simulink model "ECM_Cell"  (R2025a)
settings: Solver=FixedStepDiscrete  StartTime=0.0  StopTime=1*dt  FixedStep=dt  RelTol=1e-3
values from neighbouring files (symbols this model uses):
  a1_tbl = [ ... (first row only)    [parameters.m]
  a2_tbl = [ ... (first row only)    [parameters.m]
  C1_tbl = [ ... (first row only)    [parameters.m]
  c1_tbl = [ ... (first row only)    [parameters.m]
  C2_tbl = [ ... (first row only)    [parameters.m]
  c2_tbl = [ ... (first row only)    [parameters.m]
  I = 2    [parameters.m]
  I_bp = [1, 2, 3, 4, 5, 6, 7, 8, 9, 10, 11, 12, 13, 14, 15, 16]    [parameters.m]
  R0_tbl = [ ... (first row only)    [parameters.m]
  R1_tbl = [ ... (first row only)    [parameters.m]
  R2_tbl = [ ... (first row only)    [parameters.m]
  SOC_bp = [0, 10, 20, 30, 40, 50, 60, 70, 80, 90, 100]    [parameters.m]
  SOC_init = 80    [parameters.m]
undefined symbols (not defined in the file or in its folder): DiscIntNeverNeededParam
settings Model: Creator=ludvig  LastModifiedBy=ludvig

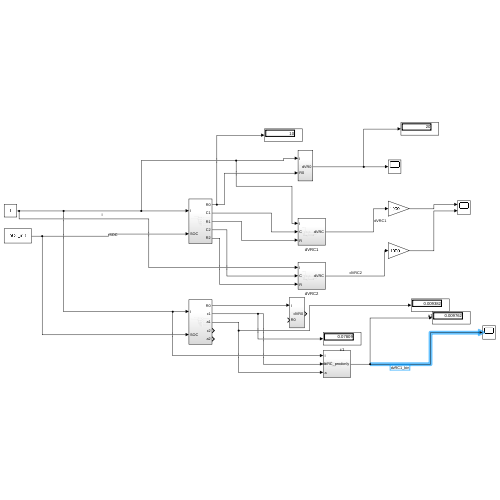
[thumbnail: Simulink's stored preview of the top-level diagram]
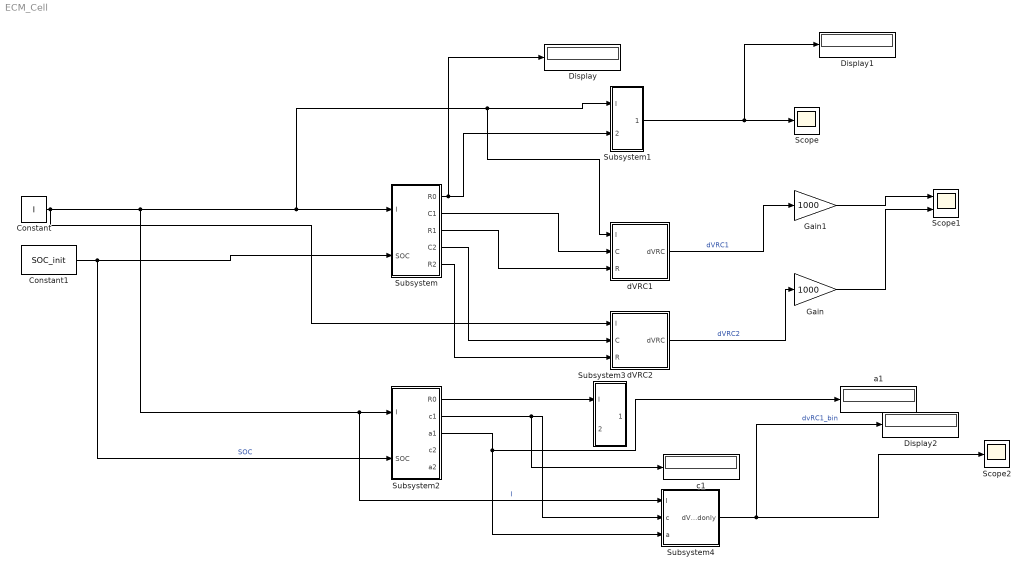
== system ECM_Cell ==
  Constant : Constant  Value=I
  Constant1 : Constant  Value=SOC_init
  Display : Display
  Display1 : Display
  Display2 : Display
  Gain : Gain  Gain=1000
  Gain1 : Gain  Gain=1000
  Scope : Scope
      settings: ActiveDisplayYMinimum=10  ActiveDisplayYMaximum=30
  Scope1 : Scope  NumInputPorts=2
      settings: ActiveDisplayYMinimum=7.0775458763666457  ActiveDisplayYMaximum=30.641709754209629
  Scope2 : Scope
      settings: ActiveDisplayYMinimum=-0.0012202262878417967  ActiveDisplayYMaximum=0.010982036590576172  DataLoggingVariableName=ScopeData2
  Subsystem : Subsystem
  Subsystem1 : Subsystem
  Subsystem2 : Subsystem
  Subsystem3 : Subsystem
  Subsystem4 : Subsystem
  a1 : Display
  c1 : Display
  dVRC1 : Subsystem
  dVRC2 : Subsystem
  wires:
  Constant/1 -> dVRC2/1(I), Subsystem4/1(I), Subsystem2/1(I), dVRC1/1(I), Subsystem1/1(I), Subsystem/1(I)  "I"
  Constant1/1 -> Subsystem2/2(SOC), Subsystem/2(SOC)  "SOC"
  Subsystem/1(R0) -> Display/1, Subsystem1/2(R0)
  Subsystem1/1(dVR0) -> Display1/1, Scope/1
  Subsystem/2(C1) -> dVRC1/2(C)
  Subsystem/3(R1) -> dVRC1/3(R)
  dVRC1/1(dVRC) -> Gain1/1  "dVRC1"
  Subsystem/4(C2) -> dVRC2/2(C)
  Subsystem/5(R2) -> dVRC2/3(R)
  dVRC2/1(dVRC) -> Gain/1  "dVRC2"
  Gain/1 -> Scope1/2
  Gain1/1 -> Scope1/1
  Subsystem2/1(R0) -> Subsystem3/1(I)
  Subsystem2/2(c1) -> c1/1, Subsystem4/2(c)
  Subsystem2/3(a1) -> a1/1, Subsystem4/3(a)
  Subsystem4/1(dVRC_prodonly) -> Display2/1, Scope2/1  "dvRC1_bin"

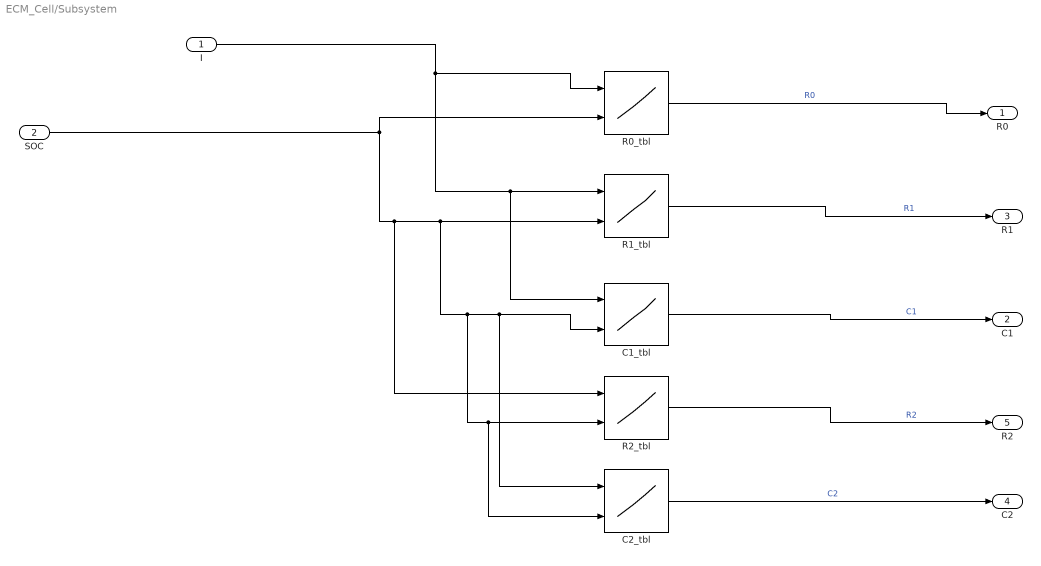
== system ECM_Cell/Subsystem ==
  I : Inport
  SOC : Inport  Port=2
  C1_tbl : Lookup_n-D  BreakpointsForDimension1=I_bp  BreakpointsForDimension2=SOC_bp  Table=C1_tbl  InternalRulePriority=Speed  RndMeth=Simplest
      settings: InputPortMap=u0,u1
  C2_tbl : Lookup_n-D  BreakpointsForDimension1=I_bp  BreakpointsForDimension2=SOC_bp  Table=C2_tbl  InternalRulePriority=Speed  RndMeth=Simplest
      settings: InputPortMap=u0,u1
  R0_tbl : Lookup_n-D  BreakpointsForDimension1=I_bp  BreakpointsForDimension2=SOC_bp  Table=R0_tbl  InternalRulePriority=Speed  RndMeth=Simplest
      settings: InputPortMap=u0,u1
  R1_tbl : Lookup_n-D  BreakpointsForDimension1=I_bp  BreakpointsForDimension2=SOC_bp  Table=R1_tbl  InternalRulePriority=Speed  RndMeth=Simplest
      settings: InputPortMap=u0,u1
  R2_tbl : Lookup_n-D  BreakpointsForDimension1=I_bp  BreakpointsForDimension2=SOC_bp  Table=R2_tbl  InternalRulePriority=Speed  RndMeth=Simplest
      settings: InputPortMap=u0,u1
  R0 : Outport
  C1 : Outport  Port=2
  R1 : Outport  Port=3
  C2 : Outport  Port=4
  R2 : Outport  Port=5
  wires:
  I/1 -> C1_tbl/1, R1_tbl/1, R0_tbl/1
  SOC/1 -> R2_tbl/1, C2_tbl/2, R2_tbl/2, C2_tbl/1, C1_tbl/2, R1_tbl/2, R0_tbl/2
  C1_tbl/1 -> C1/1  "C1"
  C2_tbl/1 -> C2/1  "C2"
  R0_tbl/1 -> R0/1  "R0"
  R2_tbl/1 -> R2/1  "R2"
  R1_tbl/1 -> R1/1  "R1"

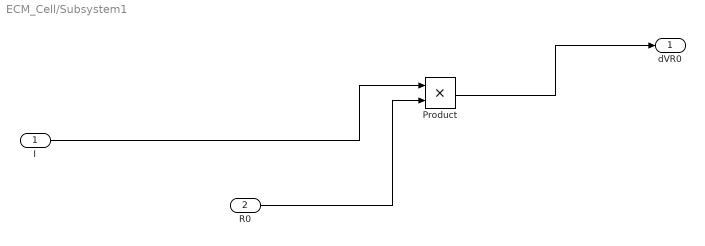
== system ECM_Cell/Subsystem1 ==
  I : Inport
  R0 : Inport  Port=2
  Product : Product
  dVR0 : Outport
  wires:
  Product/1 -> dVR0/1
  I/1 -> Product/1
  R0/1 -> Product/2

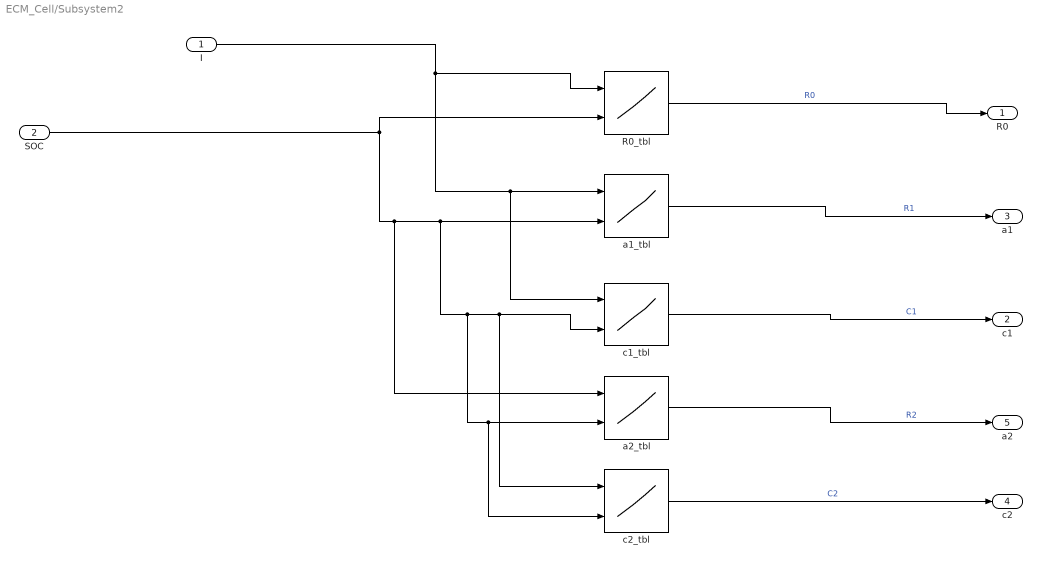
== system ECM_Cell/Subsystem2 ==
  I : Inport
  SOC : Inport  Port=2
  R0_tbl : Lookup_n-D  BreakpointsForDimension1=I_bp  BreakpointsForDimension2=SOC_bp  Table=R0_tbl  InternalRulePriority=Speed  RndMeth=Simplest
      settings: InputPortMap=u0,u1
  a1_tbl : Lookup_n-D  BreakpointsForDimension1=I_bp  BreakpointsForDimension2=SOC_bp  Table=a1_tbl  InternalRulePriority=Speed  RndMeth=Simplest
      settings: InputPortMap=u0,u1
  a2_tbl : Lookup_n-D  BreakpointsForDimension1=I_bp  BreakpointsForDimension2=SOC_bp  Table=a2_tbl  InternalRulePriority=Speed  RndMeth=Simplest
      settings: InputPortMap=u0,u1
  c1_tbl : Lookup_n-D  BreakpointsForDimension1=I_bp  BreakpointsForDimension2=SOC_bp  Table=c1_tbl  InternalRulePriority=Speed  RndMeth=Simplest
      settings: InputPortMap=u0,u1
  c2_tbl : Lookup_n-D  BreakpointsForDimension1=I_bp  BreakpointsForDimension2=SOC_bp  Table=c2_tbl  InternalRulePriority=Speed  RndMeth=Simplest
      settings: InputPortMap=u0,u1
  R0 : Outport
  c1 : Outport  Port=2
  a1 : Outport  Port=3
  c2 : Outport  Port=4
  a2 : Outport  Port=5
  wires:
  I/1 -> c1_tbl/1, a1_tbl/1, R0_tbl/1
  SOC/1 -> a2_tbl/1, c2_tbl/2, a2_tbl/2, c2_tbl/1, c1_tbl/2, a1_tbl/2, R0_tbl/2
  c1_tbl/1 -> c1/1  "C1"
  c2_tbl/1 -> c2/1  "C2"
  R0_tbl/1 -> R0/1  "R0"
  a2_tbl/1 -> a2/1  "R2"
  a1_tbl/1 -> a1/1  "R1"

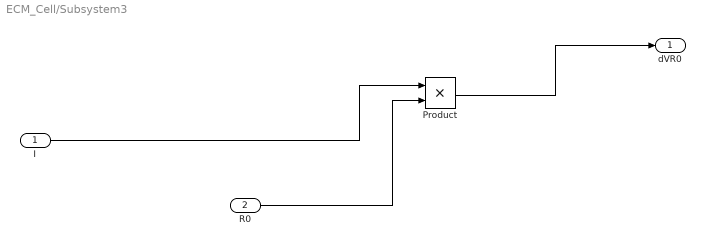
== system ECM_Cell/Subsystem3 ==
  I : Inport
  R0 : Inport  Port=2
  Product : Product
  dVR0 : Outport
  wires:
  Product/1 -> dVR0/1
  I/1 -> Product/1
  R0/1 -> Product/2

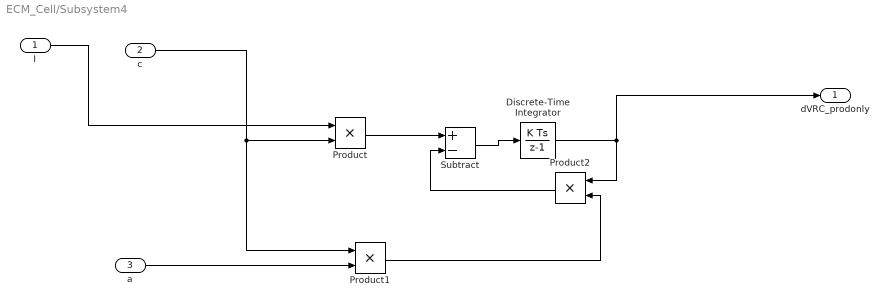
== system ECM_Cell/Subsystem4 ==
  I : Inport
  c : Inport  Port=2
  a : Inport  Port=3
  Discrete-Time Integrator : DiscreteIntegrator  SampleTime=-1  ICPrevOutput=DiscIntNeverNeededParam  ICPrevScaledInput=DiscIntNeverNeededParam
  Product : Product
  Product1 : Product
  Product2 : Product
  Subtract : Sum  Inputs=+-
  dVRC_prodonly : Outport
  wires:
  a/1 -> Product1/2
  Subtract/1 -> Discrete-Time Integrator/1
  I/1 -> Product/1
  Product2/1 -> Subtract/2
  Discrete-Time Integrator/1 -> dVRC_prodonly/1, Product2/1
  Product1/1 -> Product2/2
  Product/1 -> Subtract/1
  c/1 -> Product/2, Product1/1

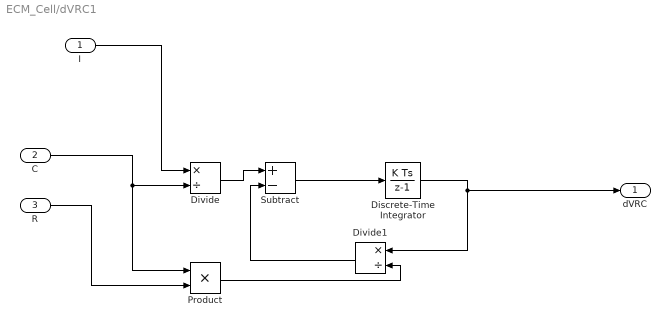
== system ECM_Cell/dVRC1 ==
  I : Inport
  C : Inport  Port=2
  R : Inport  Port=3
  Discrete-Time Integrator : DiscreteIntegrator  SampleTime=-1  ICPrevOutput=DiscIntNeverNeededParam  ICPrevScaledInput=DiscIntNeverNeededParam
  Divide : Product  Inputs=*/
  Divide1 : Product  Inputs=*/
  Product : Product
  Subtract : Sum  Inputs=+-
  dVRC : Outport
  wires:
  Divide1/1 -> Subtract/2
  Divide/1 -> Subtract/1
  I/1 -> Divide/1
  Subtract/1 -> Discrete-Time Integrator/1
  Product/1 -> Divide1/2
  R/1 -> Product/2
  C/1 -> Product/1, Divide/2
  Discrete-Time Integrator/1 -> dVRC/1, Divide1/1

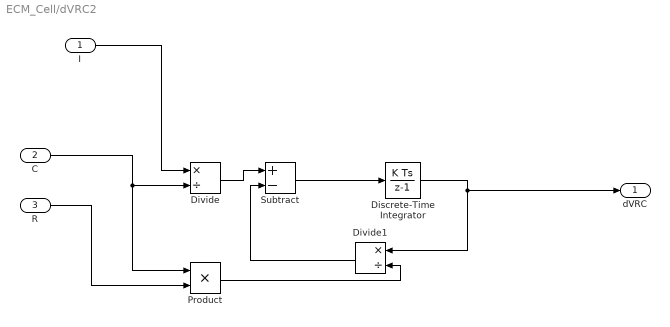
== system ECM_Cell/dVRC2 ==
  I : Inport
  C : Inport  Port=2
  R : Inport  Port=3
  Discrete-Time Integrator : DiscreteIntegrator  SampleTime=-1  ICPrevOutput=DiscIntNeverNeededParam  ICPrevScaledInput=DiscIntNeverNeededParam
  Divide : Product  Inputs=*/
  Divide1 : Product  Inputs=*/
  Product : Product
  Subtract : Sum  Inputs=+-
  dVRC : Outport
  wires:
  Divide1/1 -> Subtract/2
  Divide/1 -> Subtract/1
  I/1 -> Divide/1
  Subtract/1 -> Discrete-Time Integrator/1
  Product/1 -> Divide1/2
  R/1 -> Product/2
  C/1 -> Product/1, Divide/2
  Discrete-Time Integrator/1 -> dVRC/1, Divide1/1
